simulink model "model_spool"  (R2019b)
settings: Solver=VariableStepAuto  StartTime=0.0  StopTime=10.0  RelTol=1e-3
settings Model: Creator=artof  LastModifiedBy=artof

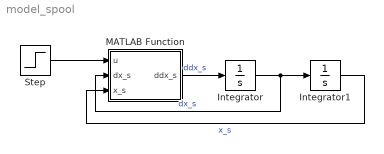
== system model_spool ==
  Integrator : Integrator
  Integrator1 : Integrator
  MATLAB Function : MATLAB Function  TreatAsAtomicUnit=on
  Step : Step  SampleTime=0
  wires:
  MATLAB Function/1(ddx_s) -> Integrator/1  "ddx_s"
  Integrator/1 -> MATLAB Function/2(dx_s), Integrator1/1  "dx_s"
  Integrator1/1 -> MATLAB Function/3(x_s)  "x_s"
  Step/1 -> MATLAB Function/1(u)

== matlab function model_spool/MATLAB Function ==
  data: u input; ddx_s output; dx_s input; x_s input
function ddx_s = fcn(u, dx_s, x_s)
ddx_s = 1 * u - 10*dx_s - 100*x_s;
ddx_s = u;
